simulink model "LIVA_AUV_SIMULATOR"  (R2023b)
settings: Solver=ode4  StartTime=0.0  StopTime=100  FixedStep=0.001  RelTol=0.01  EnableMultiTasking=on
InitFcn:
  | LIVA_AUV_Simulator_init;
model workspace (MAT data in the model file):
  a = 0.0768559116543
  a1 = 5.09287831845
  b = 2.78447714902
  b1 = 0.0150573456987
  c = 0.222680447107
  c1 = 0.0244981849866
  d = 1.17025942432
  d1 = -0.121090969634
  e = 4
  e1 = -0.000744741765672
  f = 3.22045295126
  f1 = 0.147531958158
  g = 3
  g1 = 9.31921319068e-05
  h = 4
  h1 = -0.000787888183232
  i = 2.39426372075
  i1 = -0.0976897881188
  j = 3
  j1 = 7.29765081481
  k = 2
  k1 = 3.34164431501
  l = -0.0819081975806
  l1 = 4.85550524224
  m = -0.0907196254339
  m1 = 2.91684244028
  n = 1.20537954163
  n1 = 9.00648148706
  o = 1.92822193114
  o1 = 2.79427167815
  p = 1.9547800679
  p1 = 9.64465760947
  r = 2
  r1 = 9.85880905818
  s = 0.00182097897058
  s1 = 6.72892013716
values from neighbouring files (symbols this model uses):
  alfa = 1.1    [LIVA_AUV_Simulator_init.m]
  B = 114.8*pk    (= 149.24)    [LIVA_AUV_Simulator_init.m]
  Hybrid_pKd = 1.9282219311449538    (= 1.92822193114)    [LIVA_AUV_Simulator_init.m]
  Hybrid_pKi = 1.205379541632126    (= 1.20537954163)    [LIVA_AUV_Simulator_init.m]
  Hybrid_pKp = -0.090719625433908213    (= -0.0907196254339)    [LIVA_AUV_Simulator_init.m]
  Hybrid_rKd = -0.0819081975805605    (= -0.0819081975806)    [LIVA_AUV_Simulator_init.m]
  Hybrid_rKi = 2    [LIVA_AUV_Simulator_init.m]
  Hybrid_rKp = 3    [LIVA_AUV_Simulator_init.m]
  Hybrid_xalfa = 5.092878318451735    (= 5.09287831845)    [LIVA_AUV_Simulator_init.m]
  Hybrid_xbeta = 0.024498184986623803    (= 0.0244981849866)    [LIVA_AUV_Simulator_init.m]
  Hybrid_xKd = 0.22268044710682114    (= 0.222680447107)    [LIVA_AUV_Simulator_init.m]
  Hybrid_xKi = 2.7844771490230995    (= 2.78447714902)    [LIVA_AUV_Simulator_init.m]
  Hybrid_xKp = 0.076855911654313547    (= 0.0768559116543)    [LIVA_AUV_Simulator_init.m]
  Hybrid_yalfa = -0.12109096963388193    (= -0.121090969634)    [LIVA_AUV_Simulator_init.m]
  Hybrid_ybeta = 0.14753195815811565    (= 0.147531958158)    [LIVA_AUV_Simulator_init.m]
  Hybrid_yKd = 3.2204529512582094    (= 3.22045295126)    [LIVA_AUV_Simulator_init.m]
  Hybrid_yKi = 4    [LIVA_AUV_Simulator_init.m]
  Hybrid_yKp = 1.1702594243169564    (= 1.17025942432)    [LIVA_AUV_Simulator_init.m]
  Hybrid_ywKd = 0.001820978970578287    (= 0.00182097897058)    [LIVA_AUV_Simulator_init.m]
  Hybrid_ywKi = 2    [LIVA_AUV_Simulator_init.m]
  Hybrid_ywKp = 1.9547800678980167    (= 1.9547800679)    [LIVA_AUV_Simulator_init.m]
  Hybrid_zalfa = 0.000093192131906777681    (= 9.31921319068e-05)    [LIVA_AUV_Simulator_init.m]
  Hybrid_zbeta = -0.097689788118772547    (= -0.0976897881188)    [LIVA_AUV_Simulator_init.m]
  Hybrid_zKd = 2.3942637207502    (= 2.39426372075)    [LIVA_AUV_Simulator_init.m]
  Hybrid_zKi = 4    [LIVA_AUV_Simulator_init.m]
  Hybrid_zKp = 3    [LIVA_AUV_Simulator_init.m]
  iPID_pKd = 0.00013750228463629022    (= 0.000137502284636)    [LIVA_AUV_Simulator_init.m]
  iPID_pKi = 0.031254576821627369    (= 0.0312545768216)    [LIVA_AUV_Simulator_init.m]
  iPID_pKp = 0    [LIVA_AUV_Simulator_init.m]
  iPID_rKd = 2    [LIVA_AUV_Simulator_init.m]
  iPID_rKi = 9.65529148649622E-19    (= 9.6552914865e-19)    [LIVA_AUV_Simulator_init.m]
  iPID_rKp = 3    [LIVA_AUV_Simulator_init.m]
  iPID_xKd = 0    [LIVA_AUV_Simulator_init.m]
  iPID_xKi = 1.1219546659293831    (= 1.12195466593)    [LIVA_AUV_Simulator_init.m]
  iPID_xKp = 0.018002365678869262    (= 0.0180023656789)    [LIVA_AUV_Simulator_init.m]
  iPID_yKd = 3.4277809029094881E-18    (= 3.42778090291e-18)    [LIVA_AUV_Simulator_init.m]
  iPID_yKi = 0.13401348623396903    (= 0.134013486234)    [LIVA_AUV_Simulator_init.m]
  iPID_yKp = 3    [LIVA_AUV_Simulator_init.m]
  iPID_ywKd = 0.62280020767048139    (= 0.62280020767)    [LIVA_AUV_Simulator_init.m]
  iPID_ywKi = 2    [LIVA_AUV_Simulator_init.m]
  iPID_ywKp = 0.87058892280816969    (= 0.870588922808)    [LIVA_AUV_Simulator_init.m]
  iPID_zKd = 0.00075053756185264819    (= 0.000750537561853)    [LIVA_AUV_Simulator_init.m]
  iPID_zKi = 3.5484685597653076    (= 3.54846855977)    [LIVA_AUV_Simulator_init.m]
  iPID_zKp = 0.26825539985723995    (= 0.268255399857)    [LIVA_AUV_Simulator_init.m]
  Ix = 0.16*pk    (= 0.208)    [LIVA_AUV_Simulator_init.m]
  Iy = 0.16*pk    (= 0.208)    [LIVA_AUV_Simulator_init.m]
  Iz = 0.16*pk    (= 0.208)    [LIVA_AUV_Simulator_init.m]
  Kc = 20*eye(6)    [LIVA_AUV_Simulator_init.m]
  Kp = 11.7*pk    (= 15.21)    [LIVA_AUV_Simulator_init.m]
  Kpdot = 0*pk    (= 0)    [LIVA_AUV_Simulator_init.m]
  Kpp = 1.55*pk    (= 2.015)    [LIVA_AUV_Simulator_init.m]
  Mq = 15*pk    (= 19.5)    [LIVA_AUV_Simulator_init.m]
  Mqdot = 0.0023*pk    (= 0.00299)    [LIVA_AUV_Simulator_init.m]
  Mqq = 1.55*pk    (= 2.015)    [LIVA_AUV_Simulator_init.m]
  Nr = 30*pk    (= 39)    [LIVA_AUV_Simulator_init.m]
  Nrdot = 0.0023*pk    (= 0.00299)    [LIVA_AUV_Simulator_init.m]
  Nrr = 1.55*pk    (= 2.015)    [LIVA_AUV_Simulator_init.m]
  PID_pKd = -0.04940918869876651    (= -0.0494091886988)    [LIVA_AUV_Simulator_init.m]
  PID_pKi = 2    [LIVA_AUV_Simulator_init.m]
  PID_pKp = -0.39327079611315297    (= -0.393270796113)    [LIVA_AUV_Simulator_init.m]
  PID_rKd = -0.054985573360707168    (= -0.0549855733607)    [LIVA_AUV_Simulator_init.m]
  PID_rKi = 0.001    [LIVA_AUV_Simulator_init.m]
  PID_rKp = -0.040345732248197354    (= -0.0403457322482)    [LIVA_AUV_Simulator_init.m]
  PID_xKd = 4    [LIVA_AUV_Simulator_init.m]
  PID_xKi = 4    [LIVA_AUV_Simulator_init.m]
  PID_xKp = 3    [LIVA_AUV_Simulator_init.m]
  PID_yKd = 3.1154066328676535    (= 3.11540663287)    [LIVA_AUV_Simulator_init.m]
  PID_yKi = 4    [LIVA_AUV_Simulator_init.m]
  PID_yKp = 3    [LIVA_AUV_Simulator_init.m]
  PID_ywKd = 0.89665765450717427    (= 0.896657654507)    [LIVA_AUV_Simulator_init.m]
  PID_ywKi = -0.006253695766722793    (= -0.00625369576672)    [LIVA_AUV_Simulator_init.m]
  PID_ywKp = 0.98566932171151178    (= 0.985669321712)    [LIVA_AUV_Simulator_init.m]
  PID_zKd = 0.01813689620732389    (= 0.0181368962073)    [LIVA_AUV_Simulator_init.m]
  PID_zKi = 4    [LIVA_AUV_Simulator_init.m]
  PID_zKp = 3    [LIVA_AUV_Simulator_init.m]
  Tmax = 40    [LIVA_AUV_Simulator_init.m]
  Ts_controller = 0.001    [LIVA_AUV_Simulator_init.m]
  twodof_palfa = 0.25    [LIVA_AUV_Simulator_init.m]
  twodof_pbeta = 0.12    [LIVA_AUV_Simulator_init.m]
  twodof_pKd = 0.095424714936744218    (= 0.0954247149367)    [LIVA_AUV_Simulator_init.m]
  twodof_pKi = 0.13825854798036114    (= 0.13825854798)    [LIVA_AUV_Simulator_init.m]
  twodof_pKp = 0.11369893762575015    (= 0.113698937626)    [LIVA_AUV_Simulator_init.m]
  twodof_ralfa = 0.19999999999999798    (= 0.2)    [LIVA_AUV_Simulator_init.m]
  twodof_rbeta = 0.20000000000000065    (= 0.2)    [LIVA_AUV_Simulator_init.m]
  twodof_rKd = 0.53578437965746184    (= 0.535784379657)    [LIVA_AUV_Simulator_init.m]
  twodof_rKi = 1.1506401605012322    (= 1.1506401605)    [LIVA_AUV_Simulator_init.m]
  twodof_rKp = 2.9999790377213507    (= 2.99997903772)    [LIVA_AUV_Simulator_init.m]
  twodof_xalfa = 0.30234710594262    (= 0.302347105943)    [LIVA_AUV_Simulator_init.m]
  twodof_xbeta = 1.7366690704427536    (= 1.73666907044)    [LIVA_AUV_Simulator_init.m]
  twodof_xKd = 0.97271920084965735    (= 0.97271920085)    [LIVA_AUV_Simulator_init.m]
  twodof_xKi = 3.9943078181304963    (= 3.99430781813)    [LIVA_AUV_Simulator_init.m]
  twodof_xKp = 0.28411216909151349    (= 0.284112169092)    [LIVA_AUV_Simulator_init.m]
  twodof_yalfa = 0.10435250246875363    (= 0.104352502469)    [LIVA_AUV_Simulator_init.m]
  twodof_ybeta = 0.005650227565256156    (= 0.00565022756526)    [LIVA_AUV_Simulator_init.m]
  twodof_yKd = 0.18997113533365648    (= 0.189971135334)    [LIVA_AUV_Simulator_init.m]
  twodof_yKi = 3.9999790377213498    (= 3.99997903772)    [LIVA_AUV_Simulator_init.m]
  twodof_yKp = 0.063666271676642031    (= 0.0636662716766)    [LIVA_AUV_Simulator_init.m]
  twodof_ywalfa = -4.2798991350061177    (= -4.27989913501)    [LIVA_AUV_Simulator_init.m]
  twodof_ywbeta = 0.35373480857737255    (= 0.353734808577)    [LIVA_AUV_Simulator_init.m]
  twodof_ywKd = 1.0659867557210738    (= 1.06598675572)    [LIVA_AUV_Simulator_init.m]
  twodof_ywKi = 0.00008440390384513819    (= 8.44039038451e-05)    [LIVA_AUV_Simulator_init.m]
  twodof_ywKp = 0.28527888951964514    (= 0.28527888952)    [LIVA_AUV_Simulator_init.m]
  twodof_zalfa = 0.00008034865340691478    (= 8.03486534069e-05)    [LIVA_AUV_Simulator_init.m]
  twodof_zbeta = 0.32801506093302246    (= 0.328015060933)    [LIVA_AUV_Simulator_init.m]
  twodof_zKd = 2.2289396936947683    (= 2.22893969369)    [LIVA_AUV_Simulator_init.m]
  twodof_zKi = 3.8840765857077431    (= 3.88407658571)    [LIVA_AUV_Simulator_init.m]
  twodof_zKp = 2.9999790377213507    (= 2.99997903772)    [LIVA_AUV_Simulator_init.m]
  W = 112.8*pk    (= 146.64)    [LIVA_AUV_Simulator_init.m]
  xb = 0    [LIVA_AUV_Simulator_init.m]
  xg = 0    [LIVA_AUV_Simulator_init.m]
  Xu = 26*pk    (= 33.8)    [LIVA_AUV_Simulator_init.m]
  Xudot = 10.6505*pk    (= 13.84565)    [LIVA_AUV_Simulator_init.m]
  Xuu = 18.18*pk    (= 23.634)    [LIVA_AUV_Simulator_init.m]
  yb = 0    [LIVA_AUV_Simulator_init.m]
  yg = 0    [LIVA_AUV_Simulator_init.m]
  Yv = 30*pk    (= 39)    [LIVA_AUV_Simulator_init.m]
  Yvdot = 11.9247*pk    (= 15.50211)    [LIVA_AUV_Simulator_init.m]
  Yvv = 21.66*pk    (= 28.158)    [LIVA_AUV_Simulator_init.m]
  zb = 0    [LIVA_AUV_Simulator_init.m]
  zg = 0.02    [LIVA_AUV_Simulator_init.m]
  ... (+3 more)
undefined symbols (not defined in the file or in its folder): DiscIntNeverNeededParam, gray, sigbuilder_block
libraries: slpidlib x29, eeGeneralControl x19, pid_lib x6, simulink x4, sim3dlib x4
(part 5 of 6)

== system LIVA_AUV_SIMULATOR/6DOF CONTROL/i-PID Controler/i-PID Controller  ==
  note: iPID Control Signals
  note: Error Signals
  Body Frame Reference Trajectory : Inport
  Error Signals : Inport  Port=2
  Body Frame Positions : Inport  Port=3
  Calculation : Subsystem
  Demux : Demux  Outputs=6
  Mux2 : Mux  Inputs=6
  PID Controller : pid_lib/PID Controller  Controller=PID  Form=Parallel  TimeDomain=Discrete-time  UseExternalTs=off  SampleTime=-1  IntegratorMethod=Forward Euler  FilterMethod=Forward Euler  ControllerParametersSource=internal  P=iPID_xKp  I=iPID_xKi  D=iPID_xKd  UseFilter=on  N=1  TunerSelectOption=Transfer Function Based (PID Tuner App)  InitialConditionSource=internal  InitialConditionForIntegrator=0  InitialConditionForFilter=0  DifferentiatorICPrevScaledInput=0  ExternalReset=none  TrackingMode=off  Kt=1  LimitOutput=on  SatLimitsSource=internal  UpperSaturationLimit=inf  LowerSaturationLimit=-inf  LinearizeAsGain=on  AntiWindupMode=back-calculation  Kb=1  POutMin=[]  POutMax=[]  IOutMin=[]  IOutMax=[]  DOutMin=[]  DOutMax=[]  NOutMin=[]  NOutMax=[]  SumOutMin=[]  SumOutMax=[]  SaturationOutMin=[]  SaturationOutMax=[]  PParamMin=[]  PParamMax=[]  IParamMin=[]  IParamMax=[]  DParamMin=[]  DParamMax=[]  NParamMin=[]  NParamMax=[]  KbParamMin=[]  KbParamMax=[]  KtParamMin=[]  KtParamMax=[]  KbOutMin=[]  KbOutMax=[]  KtOutMin=[]  KtOutMax=[]  IntegratorOutMin=[]  IntegratorOutMax=[]  FilterOutMin=[]  FilterOutMax=[]  SumI1OutMin=[]  SumI1OutMax=[]  SumI2OutMin=[]  SumI2OutMax=[]  SumI3OutMin=[]  SumI3OutMax=[]  SumI4OutMin=[]  SumI4OutMax=[]  SumDOutMin=[]  SumDOutMax=[]  DifferentiatorOutMin=[]  DifferentiatorOutMax=[]  FilterDiffOutCoefMin=[]  FilterDiffOutCoefMax=[]  ReciprocalOutMin=[]  ReciprocalOutMax=[]  SumDenOutMin=[]  SumDenOutMax=[]  SumNumOutMin=[]  SumNumOutMax=[]  DivideOutMin=[]  DivideOutMax=[]  UdiffTsProdOutMin=[]  UdiffTsProdOutMax=[]  NTsProdOutMin=[]  NTsProdOutMax=[]  UintegralTsProdOutMin=[]  UintegralTsProdOutMax=[]  UngainTsProdOutMin=[]  UngainTsProdOutMax=[]  IntegratorContinuousStateAttributes=''  IntegratorStateMustResolveToSignalObject=off  IntegratorRTWStateStorageClass=Auto  FilterContinuousStateAttributes=''  FilterStateMustResolveToSignalObject=off  FilterRTWStateStorageClass=Auto  ParallelPVariant=InternalParameters  IdealPVariant=Disabled  IVariant=InternalParameters  DVariant=InternalParameters  IntegratorVariant=Discrete  SatVariant=Enabled  AWVariant=BackCalculation  PCopyVariant=Disabled  TRVariant=Disabled  FdbkBlocksVariant=Forward  IdealPFdbkVariant=Disabled  SatFdbkVariant=Disabled  DerivativeFilterVariant=ForwardEulerFilter  NVariant=InternalParameters  NCopyVariant=Disabled  FilterICVariant=InternalICsFilter  IntegratorICVariant=InternalICs  ExternalResetVariant=Disabled  TRSumVariant=Passthrough  SumFdbkVariant=Disabled  SumVariant=Sum_PID  TsampFilterVariant=InternalTs  TsampNgainVariant=Passthrough  TsampIntegralVariant=Passthrough  ExternalSaturationOutDataTypeStr=Inherit: Same as second input
  PID Controller1 : pid_lib/PID Controller  Controller=PID  Form=Parallel  TimeDomain=Discrete-time  UseExternalTs=off  SampleTime=-1  IntegratorMethod=Forward Euler  FilterMethod=Forward Euler  ControllerParametersSource=internal  P=iPID_yKp  I=iPID_yKi  D=iPID_yKd  UseFilter=on  N=3  TunerSelectOption=Transfer Function Based (PID Tuner App)  InitialConditionSource=internal  InitialConditionForIntegrator=0  InitialConditionForFilter=0  DifferentiatorICPrevScaledInput=0  ExternalReset=none  TrackingMode=off  Kt=1  LimitOutput=on  SatLimitsSource=internal  UpperSaturationLimit=inf  LowerSaturationLimit=-inf  LinearizeAsGain=on  AntiWindupMode=back-calculation  Kb=1  POutMin=[]  POutMax=[]  IOutMin=[]  IOutMax=[]  DOutMin=[]  DOutMax=[]  NOutMin=[]  NOutMax=[]  SumOutMin=[]  SumOutMax=[]  SaturationOutMin=[]  SaturationOutMax=[]  PParamMin=[]  PParamMax=[]  IParamMin=[]  IParamMax=[]  DParamMin=[]  DParamMax=[]  NParamMin=[]  NParamMax=[]  KbParamMin=[]  KbParamMax=[]  KtParamMin=[]  KtParamMax=[]  KbOutMin=[]  KbOutMax=[]  KtOutMin=[]  KtOutMax=[]  IntegratorOutMin=[]  IntegratorOutMax=[]  FilterOutMin=[]  FilterOutMax=[]  SumI1OutMin=[]  SumI1OutMax=[]  SumI2OutMin=[]  SumI2OutMax=[]  SumI3OutMin=[]  SumI3OutMax=[]  SumI4OutMin=[]  SumI4OutMax=[]  SumDOutMin=[]  SumDOutMax=[]  DifferentiatorOutMin=[]  DifferentiatorOutMax=[]  FilterDiffOutCoefMin=[]  FilterDiffOutCoefMax=[]  ReciprocalOutMin=[]  ReciprocalOutMax=[]  SumDenOutMin=[]  SumDenOutMax=[]  SumNumOutMin=[]  SumNumOutMax=[]  DivideOutMin=[]  DivideOutMax=[]  UdiffTsProdOutMin=[]  UdiffTsProdOutMax=[]  NTsProdOutMin=[]  NTsProdOutMax=[]  UintegralTsProdOutMin=[]  UintegralTsProdOutMax=[]  UngainTsProdOutMin=[]  UngainTsProdOutMax=[]  IntegratorContinuousStateAttributes=''  IntegratorStateMustResolveToSignalObject=off  IntegratorRTWStateStorageClass=Auto  FilterContinuousStateAttributes=''  FilterStateMustResolveToSignalObject=off  FilterRTWStateStorageClass=Auto  ParallelPVariant=InternalParameters  IdealPVariant=Disabled  IVariant=InternalParameters  DVariant=InternalParameters  IntegratorVariant=Discrete  SatVariant=Enabled  AWVariant=BackCalculation  PCopyVariant=Disabled  TRVariant=Disabled  FdbkBlocksVariant=Forward  IdealPFdbkVariant=Disabled  SatFdbkVariant=Disabled  DerivativeFilterVariant=ForwardEulerFilter  NVariant=InternalParameters  NCopyVariant=Disabled  FilterICVariant=InternalICsFilter  IntegratorICVariant=InternalICs  ExternalResetVariant=Disabled  TRSumVariant=Passthrough  SumFdbkVariant=Disabled  SumVariant=Sum_PID  TsampFilterVariant=InternalTs  TsampNgainVariant=Passthrough  TsampIntegralVariant=Passthrough  ExternalSaturationOutDataTypeStr=Inherit: Same as second input
  PID Controller2 : pid_lib/PID Controller  Controller=PID  Form=Parallel  TimeDomain=Discrete-time  UseExternalTs=off  SampleTime=-1  IntegratorMethod=Forward Euler  FilterMethod=Forward Euler  ControllerParametersSource=internal  P=iPID_zKp  I=iPID_zKi  D=iPID_zKd  UseFilter=on  N=1  TunerSelectOption=Transfer Function Based (PID Tuner App)  InitialConditionSource=internal  InitialConditionForIntegrator=0  InitialConditionForFilter=0  DifferentiatorICPrevScaledInput=0  ExternalReset=none  TrackingMode=off  Kt=1  LimitOutput=on  SatLimitsSource=internal  UpperSaturationLimit=inf  LowerSaturationLimit=-inf  LinearizeAsGain=on  AntiWindupMode=back-calculation  Kb=1  POutMin=[]  POutMax=[]  IOutMin=[]  IOutMax=[]  DOutMin=[]  DOutMax=[]  NOutMin=[]  NOutMax=[]  SumOutMin=[]  SumOutMax=[]  SaturationOutMin=[]  SaturationOutMax=[]  PParamMin=[]  PParamMax=[]  IParamMin=[]  IParamMax=[]  DParamMin=[]  DParamMax=[]  NParamMin=[]  NParamMax=[]  KbParamMin=[]  KbParamMax=[]  KtParamMin=[]  KtParamMax=[]  KbOutMin=[]  KbOutMax=[]  KtOutMin=[]  KtOutMax=[]  IntegratorOutMin=[]  IntegratorOutMax=[]  FilterOutMin=[]  FilterOutMax=[]  SumI1OutMin=[]  SumI1OutMax=[]  SumI2OutMin=[]  SumI2OutMax=[]  SumI3OutMin=[]  SumI3OutMax=[]  SumI4OutMin=[]  SumI4OutMax=[]  SumDOutMin=[]  SumDOutMax=[]  DifferentiatorOutMin=[]  DifferentiatorOutMax=[]  FilterDiffOutCoefMin=[]  FilterDiffOutCoefMax=[]  ReciprocalOutMin=[]  ReciprocalOutMax=[]  SumDenOutMin=[]  SumDenOutMax=[]  SumNumOutMin=[]  SumNumOutMax=[]  DivideOutMin=[]  DivideOutMax=[]  UdiffTsProdOutMin=[]  UdiffTsProdOutMax=[]  NTsProdOutMin=[]  NTsProdOutMax=[]  UintegralTsProdOutMin=[]  UintegralTsProdOutMax=[]  UngainTsProdOutMin=[]  UngainTsProdOutMax=[]  IntegratorContinuousStateAttributes=''  IntegratorStateMustResolveToSignalObject=off  IntegratorRTWStateStorageClass=Auto  FilterContinuousStateAttributes=''  FilterStateMustResolveToSignalObject=off  FilterRTWStateStorageClass=Auto  ParallelPVariant=InternalParameters  IdealPVariant=Disabled  IVariant=InternalParameters  DVariant=InternalParameters  IntegratorVariant=Discrete  SatVariant=Enabled  AWVariant=BackCalculation  PCopyVariant=Disabled  TRVariant=Disabled  FdbkBlocksVariant=Forward  IdealPFdbkVariant=Disabled  SatFdbkVariant=Disabled  DerivativeFilterVariant=ForwardEulerFilter  NVariant=InternalParameters  NCopyVariant=Disabled  FilterICVariant=InternalICsFilter  IntegratorICVariant=InternalICs  ExternalResetVariant=Disabled  TRSumVariant=Passthrough  SumFdbkVariant=Disabled  SumVariant=Sum_PID  TsampFilterVariant=InternalTs  TsampNgainVariant=Passthrough  TsampIntegralVariant=Passthrough  ExternalSaturationOutDataTypeStr=Inherit: Same as second input
  PID Controller3 : pid_lib/PID Controller  Controller=PID  Form=Parallel  TimeDomain=Discrete-time  UseExternalTs=off  SampleTime=-1  IntegratorMethod=Forward Euler  FilterMethod=Forward Euler  ControllerParametersSource=internal  P=iPID_rKp  I=iPID_rKi  D=iPID_rKd  UseFilter=on  N=1  TunerSelectOption=Transfer Function Based (PID Tuner App)  InitialConditionSource=internal  InitialConditionForIntegrator=0  InitialConditionForFilter=0  DifferentiatorICPrevScaledInput=0  ExternalReset=none  TrackingMode=off  Kt=1  LimitOutput=on  SatLimitsSource=internal  UpperSaturationLimit=inf  LowerSaturationLimit=-inf  LinearizeAsGain=on  AntiWindupMode=back-calculation  Kb=1  POutMin=[]  POutMax=[]  IOutMin=[]  IOutMax=[]  DOutMin=[]  DOutMax=[]  NOutMin=[]  NOutMax=[]  SumOutMin=[]  SumOutMax=[]  SaturationOutMin=[]  SaturationOutMax=[]  PParamMin=[]  PParamMax=[]  IParamMin=[]  IParamMax=[]  DParamMin=[]  DParamMax=[]  NParamMin=[]  NParamMax=[]  KbParamMin=[]  KbParamMax=[]  KtParamMin=[]  KtParamMax=[]  KbOutMin=[]  KbOutMax=[]  KtOutMin=[]  KtOutMax=[]  IntegratorOutMin=[]  IntegratorOutMax=[]  FilterOutMin=[]  FilterOutMax=[]  SumI1OutMin=[]  SumI1OutMax=[]  SumI2OutMin=[]  SumI2OutMax=[]  SumI3OutMin=[]  SumI3OutMax=[]  SumI4OutMin=[]  SumI4OutMax=[]  SumDOutMin=[]  SumDOutMax=[]  DifferentiatorOutMin=[]  DifferentiatorOutMax=[]  FilterDiffOutCoefMin=[]  FilterDiffOutCoefMax=[]  ReciprocalOutMin=[]  ReciprocalOutMax=[]  SumDenOutMin=[]  SumDenOutMax=[]  SumNumOutMin=[]  SumNumOutMax=[]  DivideOutMin=[]  DivideOutMax=[]  UdiffTsProdOutMin=[]  UdiffTsProdOutMax=[]  NTsProdOutMin=[]  NTsProdOutMax=[]  UintegralTsProdOutMin=[]  UintegralTsProdOutMax=[]  UngainTsProdOutMin=[]  UngainTsProdOutMax=[]  IntegratorContinuousStateAttributes=''  IntegratorStateMustResolveToSignalObject=off  IntegratorRTWStateStorageClass=Auto  FilterContinuousStateAttributes=''  FilterStateMustResolveToSignalObject=off  FilterRTWStateStorageClass=Auto  ParallelPVariant=InternalParameters  IdealPVariant=Disabled  IVariant=InternalParameters  DVariant=InternalParameters  IntegratorVariant=Discrete  SatVariant=Enabled  AWVariant=BackCalculation  PCopyVariant=Disabled  TRVariant=Disabled  FdbkBlocksVariant=Forward  IdealPFdbkVariant=Disabled  SatFdbkVariant=Disabled  DerivativeFilterVariant=ForwardEulerFilter  NVariant=InternalParameters  NCopyVariant=Disabled  FilterICVariant=InternalICsFilter  IntegratorICVariant=InternalICs  ExternalResetVariant=Disabled  TRSumVariant=Passthrough  SumFdbkVariant=Disabled  SumVariant=Sum_PID  TsampFilterVariant=InternalTs  TsampNgainVariant=Passthrough  TsampIntegralVariant=Passthrough  ExternalSaturationOutDataTypeStr=Inherit: Same as second input
  PID Controller4 : pid_lib/PID Controller  Controller=PID  Form=Parallel  TimeDomain=Discrete-time  UseExternalTs=off  SampleTime=-1  IntegratorMethod=Forward Euler  FilterMethod=Forward Euler  ControllerParametersSource=internal  P=iPID_pKp  I=iPID_pKi  D=iPID_pKd  UseFilter=on  N=1  TunerSelectOption=Transfer Function Based (PID Tuner App)  InitialConditionSource=internal  InitialConditionForIntegrator=0  InitialConditionForFilter=0  DifferentiatorICPrevScaledInput=0  ExternalReset=none  TrackingMode=off  Kt=1  LimitOutput=on  SatLimitsSource=internal  UpperSaturationLimit=inf  LowerSaturationLimit=-inf  LinearizeAsGain=on  AntiWindupMode=back-calculation  Kb=1  POutMin=[]  POutMax=[]  IOutMin=[]  IOutMax=[]  DOutMin=[]  DOutMax=[]  NOutMin=[]  NOutMax=[]  SumOutMin=[]  SumOutMax=[]  SaturationOutMin=[]  SaturationOutMax=[]  PParamMin=[]  PParamMax=[]  IParamMin=[]  IParamMax=[]  DParamMin=[]  DParamMax=[]  NParamMin=[]  NParamMax=[]  KbParamMin=[]  KbParamMax=[]  KtParamMin=[]  KtParamMax=[]  KbOutMin=[]  KbOutMax=[]  KtOutMin=[]  KtOutMax=[]  IntegratorOutMin=[]  IntegratorOutMax=[]  FilterOutMin=[]  FilterOutMax=[]  SumI1OutMin=[]  SumI1OutMax=[]  SumI2OutMin=[]  SumI2OutMax=[]  SumI3OutMin=[]  SumI3OutMax=[]  SumI4OutMin=[]  SumI4OutMax=[]  SumDOutMin=[]  SumDOutMax=[]  DifferentiatorOutMin=[]  DifferentiatorOutMax=[]  FilterDiffOutCoefMin=[]  FilterDiffOutCoefMax=[]  ReciprocalOutMin=[]  ReciprocalOutMax=[]  SumDenOutMin=[]  SumDenOutMax=[]  SumNumOutMin=[]  SumNumOutMax=[]  DivideOutMin=[]  DivideOutMax=[]  UdiffTsProdOutMin=[]  UdiffTsProdOutMax=[]  NTsProdOutMin=[]  NTsProdOutMax=[]  UintegralTsProdOutMin=[]  UintegralTsProdOutMax=[]  UngainTsProdOutMin=[]  UngainTsProdOutMax=[]  IntegratorContinuousStateAttributes=''  IntegratorStateMustResolveToSignalObject=off  IntegratorRTWStateStorageClass=Auto  FilterContinuousStateAttributes=''  FilterStateMustResolveToSignalObject=off  FilterRTWStateStorageClass=Auto  ParallelPVariant=InternalParameters  IdealPVariant=Disabled  IVariant=InternalParameters  DVariant=InternalParameters  IntegratorVariant=Discrete  SatVariant=Enabled  AWVariant=BackCalculation  PCopyVariant=Disabled  TRVariant=Disabled  FdbkBlocksVariant=Forward  IdealPFdbkVariant=Disabled  SatFdbkVariant=Disabled  DerivativeFilterVariant=ForwardEulerFilter  NVariant=InternalParameters  NCopyVariant=Disabled  FilterICVariant=InternalICsFilter  IntegratorICVariant=InternalICs  ExternalResetVariant=Disabled  TRSumVariant=Passthrough  SumFdbkVariant=Disabled  SumVariant=Sum_PID  TsampFilterVariant=InternalTs  TsampNgainVariant=Passthrough  TsampIntegralVariant=Passthrough  ExternalSaturationOutDataTypeStr=Inherit: Same as second input
  PID Controller5 : pid_lib/PID Controller  Controller=PID  Form=Parallel  TimeDomain=Discrete-time  UseExternalTs=off  SampleTime=-1  IntegratorMethod=Forward Euler  FilterMethod=Forward Euler  ControllerParametersSource=internal  P=iPID_ywKp  I=iPID_ywKi  D=iPID_ywKd  UseFilter=on  N=1  TunerSelectOption=Transfer Function Based (PID Tuner App)  InitialConditionSource=internal  InitialConditionForIntegrator=0  InitialConditionForFilter=0  DifferentiatorICPrevScaledInput=0  ExternalReset=none  TrackingMode=off  Kt=1  LimitOutput=on  SatLimitsSource=internal  UpperSaturationLimit=inf  LowerSaturationLimit=-inf  LinearizeAsGain=on  AntiWindupMode=back-calculation  Kb=1  POutMin=[]  POutMax=[]  IOutMin=[]  IOutMax=[]  DOutMin=[]  DOutMax=[]  NOutMin=[]  NOutMax=[]  SumOutMin=[]  SumOutMax=[]  SaturationOutMin=[]  SaturationOutMax=[]  PParamMin=[]  PParamMax=[]  IParamMin=[]  IParamMax=[]  DParamMin=[]  DParamMax=[]  NParamMin=[]  NParamMax=[]  KbParamMin=[]  KbParamMax=[]  KtParamMin=[]  KtParamMax=[]  KbOutMin=[]  KbOutMax=[]  KtOutMin=[]  KtOutMax=[]  IntegratorOutMin=[]  IntegratorOutMax=[]  FilterOutMin=[]  FilterOutMax=[]  SumI1OutMin=[]  SumI1OutMax=[]  SumI2OutMin=[]  SumI2OutMax=[]  SumI3OutMin=[]  SumI3OutMax=[]  SumI4OutMin=[]  SumI4OutMax=[]  SumDOutMin=[]  SumDOutMax=[]  DifferentiatorOutMin=[]  DifferentiatorOutMax=[]  FilterDiffOutCoefMin=[]  FilterDiffOutCoefMax=[]  ReciprocalOutMin=[]  ReciprocalOutMax=[]  SumDenOutMin=[]  SumDenOutMax=[]  SumNumOutMin=[]  SumNumOutMax=[]  DivideOutMin=[]  DivideOutMax=[]  UdiffTsProdOutMin=[]  UdiffTsProdOutMax=[]  NTsProdOutMin=[]  NTsProdOutMax=[]  UintegralTsProdOutMin=[]  UintegralTsProdOutMax=[]  UngainTsProdOutMin=[]  UngainTsProdOutMax=[]  IntegratorContinuousStateAttributes=''  IntegratorStateMustResolveToSignalObject=off  IntegratorRTWStateStorageClass=Auto  FilterContinuousStateAttributes=''  FilterStateMustResolveToSignalObject=off  FilterRTWStateStorageClass=Auto  ParallelPVariant=InternalParameters  IdealPVariant=Disabled  IVariant=InternalParameters  DVariant=InternalParameters  IntegratorVariant=Discrete  SatVariant=Enabled  AWVariant=BackCalculation  PCopyVariant=Disabled  TRVariant=Disabled  FdbkBlocksVariant=Forward  IdealPFdbkVariant=Disabled  SatFdbkVariant=Disabled  DerivativeFilterVariant=ForwardEulerFilter  NVariant=InternalParameters  NCopyVariant=Disabled  FilterICVariant=InternalICsFilter  IntegratorICVariant=InternalICs  ExternalResetVariant=Disabled  TRSumVariant=Passthrough  SumFdbkVariant=Disabled  SumVariant=Sum_PID  TsampFilterVariant=InternalTs  TsampNgainVariant=Passthrough  TsampIntegralVariant=Passthrough  ExternalSaturationOutDataTypeStr=Inherit: Same as second input
  iPID Control Signals : Outport  VectorParamsAs1DForOutWhenUnconnected=off
  wires:
  Body Frame Reference Trajectory/1 -> Calculation/1(Body Frame Reference Trajectory)
  Body Frame Positions/1 -> Calculation/3(Body Frame Positions)
  Calculation/1(IPI Controller Outputs) -> iPID Control Signals/1
  PID Controller3/1 -> Mux2/4
  Error Signals/1 -> Demux/1
  Demux/5 -> PID Controller4/1
  PID Controller2/1 -> Mux2/3
  PID Controller1/1 -> Mux2/2
  Demux/4 -> PID Controller3/1
  Demux/1 -> PID Controller/1
  Mux2/1 -> Calculation/2(PI Controller Outputs)  "PI Controller Outputs"
  PID Controller5/1 -> Mux2/6
  PID Controller4/1 -> Mux2/5
  Demux/3 -> PID Controller2/1
  Demux/2 -> PID Controller1/1
  Demux/6 -> PID Controller5/1
  PID Controller/1 -> Mux2/1

== system LIVA_AUV_SIMULATOR/Evaluation & Visualization/Variant Subsystem/3D Unreal Engine ==
  Visualization : Inport
  Constant : Constant  Value=[1 1 1]
  Demux : Demux  Outputs=2
  Simulation 3D Actor Transform Set : sim3dlib/Simulation 3D Actor Transform Set  Priority=-1  ActorTag=Sub1  NumberOfParts=1  CustNumOfParts=3  Translation=[0 0 0]  Rotation=[0 0 0]  Scale=[1 1 1]  Ts=-1  aMode=2
  Simulation 3D Camera Get : sim3dlib/Simulation 3D Camera Get  Priority=1  sensorTag=Sim3dSensor3  sensorId=3  sensorName=Sim3dSensor3  vehTagList={'Scene Origin'}  vehTag=Scene Origin  mountLoc=Origin  offsetFlag=on  tmountOffset=[6.5, 13.5, 12]  rmountOffset=[0, 28, 225]  HorizontalResolution=1280  VerticalResolution=720  HorizontalFOV=60  SampleTime=-1  mountPoint=[6.5 -13.5 12]  mountOrientation=[0 -28 -225]  aMode=2  ID=3
  Simulation 3D Scene Configuration : sim3dlib/Simulation 3D Scene Configuration  Priority=0  ProjectFormat=Unreal Editor  SceneDesc=Straight road  ProjectName=C:\MATLAB\toolbox\shared\sim3d_projects\automotive_project\UE4\WindowsNoEditor\VehicleSimulation.exe  ScenePath=/Game/Maps/HwStrght  UEProjPath=D:\UE\projects\MyProject77\MyProject77.uproject  EnableOpenDRIVE=off  vehTagList={'Scene Origin'}  vehTag=Scene Origin  OpVisEn=off  Ts=0.01  EnableWindow=on  EnableRemoteAccess=off  EnableWeather=off  SunAltitude=40.0  SunAzimuth=90  clouds=10  wind=1  fog=0  rain=0  EnableGeospatial=off  OriginHeight=200  OriginLatitude=40.744652  OriginLongitude=-73.988864  MapStyle=Aerial  AdditionalAssetIDs=[]  UseAdvancedSunSky=off  SolarTime=11  TimeZone=-5  Day=21  Month=9  Year=2022  UseDaylightSavingTime=on  DSTStartDay=10  DSTStartMonth=3  DSTEndDay=3  DSTEndMonth=11  DSTSwitchHour=2  sensorTag=MainCamera1  sensorId=1  sensorName=MainCamera1  mountLoc=Origin  offsetFlag=off  tmountOffset=[0, 0, 0]  rmountOffset=[0, 0, 0]  HorizontalResolution=1280  VerticalResolution=720  HorizontalFOV=60  mountPoint=[0 0 0]  mountOrientation=[0 0 0]  aMode=2  ID=1  GeoTrigger=Inactive
  Subsystem : Subsystem
  Subsystem1 : Subsystem
  Video Viewer : VideoViewer  colormapValue=gray(256)  FigPos=[624 1037 1296 929]
  wires:
  Subsystem1/1(Out1) -> Simulation 3D Actor Transform Set/2
  Constant/1 -> Simulation 3D Actor Transform Set/3
  Demux/2 -> Subsystem1/1(In1)
  Demux/1 -> Subsystem/1(In1)
  Subsystem/1(Out1) -> Simulation 3D Actor Transform Set/1
  Simulation 3D Camera Get/1 -> Video Viewer/1
  Visualization/1 -> Demux/1

== system LIVA_AUV_SIMULATOR/Evaluation & Visualization/Variant Subsystem/Simulink Scopes ==
  Visualization : Inport

== system LIVA_AUV_SIMULATOR/6DOF CONTROL/2 DoF i-PID Controller/ i-PID Feedback Controller /Calculation ==
  Body Frame Reference Trajectory : Inport
  PI Controller Outputs : Inport  Port=2
  Body Frame Positions : Inport  Port=3
  Divide : Product  Inputs=*/
  Divide1 : Product  Inputs=**
  Divide2 : Product  Inputs=*/
  Filtered Derivative (Discrete or Continuous){,1..3} (4 alike) : eeGeneralControl/Filtered Derivative (Discrete or Continuous)  K=1  T=1  B=inf  A=-inf  minRatio=10  init_option=Inherited from block input  x0=0  Ts=-1
  Sum : Sum  Inputs=|+-
  Sum1 : Sum  Inputs=|+-
  Sum2 : Sum  Inputs=|++
  Unit Delay : UnitDelay  SampleTime=-1  HasFrameUpgradeWarning=on
  a : Constant  Value=alfa
  IPI Controller Outputs : Outport
  wires:
  a/1 -> Divide1/2, Divide/2, Divide2/2
  Divide/1 -> Sum/2
  Divide1/1 -> Sum1/2
  Sum1/1 -> Divide/1  "F"
  Unit Delay/1 -> Divide1/1
  Filtered Derivative (Discrete or Continuous)1/1 -> Sum/1
  Body Frame Reference Trajectory/1 -> Filtered Derivative (Discrete or Continuous)/1
  PI Controller Outputs/1 -> Sum2/2
  Sum/1 -> Divide2/1
  Divide2/1 -> Sum2/1
  Sum2/1 -> Unit Delay/1, IPI Controller Outputs/1
  Body Frame Positions/1 -> Filtered Derivative (Discrete or Continuous)2/1
  Filtered Derivative (Discrete or Continuous)3/1 -> Sum1/1
  Filtered Derivative (Discrete or Continuous)/1 -> Filtered Derivative (Discrete or Continuous)1/1
  Filtered Derivative (Discrete or Continuous)2/1 -> Filtered Derivative (Discrete or Continuous)3/1

== system LIVA_AUV_SIMULATOR/6DOF CONTROL/Hybrid i-PID Controller/2-DoF i-PID Position Controller/Feedback i-PID Controller  ==
  note: iPID Control Signals
  note: Error Signals
  Body Frame Reference Trajectory : Inport
  Error Signals : Inport  Port=2
  Body Frame Positions : Inport  Port=3
  Calculation : Subsystem
  Demux : Demux  Outputs=3
  Mux2 : Mux  Inputs=3
  PID Controller : slpidlib/PID Controller  Controller=PID  Form=Parallel  TimeDomain=Discrete-time  UseExternalTs=off  SampleTime=Ts_controller  IntegratorMethod=Forward Euler  FilterMethod=Forward Euler  ControllerParametersSource=internal  P=Hybrid_xKp  I=Hybrid_xKi  UseKiTs=off  D=Hybrid_xKd  N=0.8  UseFilter=on  TunerSelectOption=Transfer Function Based (PID Tuner App)  InitialConditionSource=internal  InitialConditionForIntegrator=0  InitialConditionForFilter=0  DifferentiatorICPrevScaledInput=0  ExternalReset=none  TrackingMode=off  Kt=1  LimitOutput=on  SatLimitsSource=internal  UpperSaturationLimit=inf  LowerSaturationLimit=-inf  LinearizeAsGain=on  AntiWindupMode=back-calculation  Kb=1  LimitIntegrator=off  UpperIntegratorSaturationLimit=inf  LowerIntegratorSaturationLimit=-inf  POutMin=[]  POutMax=[]  IOutMin=[]  IOutMax=[]  DOutMin=[]  DOutMax=[]  NOutMin=[]  NOutMax=[]  SumOutMin=[]  SumOutMax=[]  SaturationOutMin=[]  SaturationOutMax=[]  PParamMin=[]  PParamMax=[]  IParamMin=[]  IParamMax=[]  DParamMin=[]  DParamMax=[]  NParamMin=[]  NParamMax=[]  KbParamMin=[]  KbParamMax=[]  KtParamMin=[]  KtParamMax=[]  KbOutMin=[]  KbOutMax=[]  KtOutMin=[]  KtOutMax=[]  IntegratorOutMin=[]  IntegratorOutMax=[]  FilterOutMin=[]  FilterOutMax=[]  SumI1OutMin=[]  SumI1OutMax=[]  SumI2OutMin=[]  SumI2OutMax=[]  SumI3OutMin=[]  SumI3OutMax=[]  SumI4OutMin=[]  SumI4OutMax=[]  SumDOutMin=[]  SumDOutMax=[]  DifferentiatorOutMin=[]  DifferentiatorOutMax=[]  FilterDiffOutCoefMin=[]  FilterDiffOutCoefMax=[]  ReciprocalOutMin=[]  ReciprocalOutMax=[]  SumDenOutMin=[]  SumDenOutMax=[]  SumNumOutMin=[]  SumNumOutMax=[]  DivideOutMin=[]  DivideOutMax=[]  UdiffTsProdOutMin=[]  UdiffTsProdOutMax=[]  NTsProdOutMin=[]  NTsProdOutMax=[]  UintegralTsProdOutMin=[]  UintegralTsProdOutMax=[]  UngainTsProdOutMin=[]  UngainTsProdOutMax=[]  ClampingZeroOutDataTypeStr=Inherit: Inherit via back propagation  ClampingZeroOutMin=[]  ClampingZeroOutMax=[]  FilterDenConstantOutDataTypeStr=Inherit: Inherit via back propagation  FilterDenConstantOutMin=[]  FilterDenConstantOutMax=[]  PCopyOutDataTypeStr=Inherit: Inherit via back propagation  PCopyOutMin=[]  PCopyOutMax=[]  NCopyOutDataTypeStr=Inherit: Inherit via back propagation  NCopyOutMin=[]  NCopyOutMax=[]  IntegratorContinuousStateAttributes=''  IntegratorStateMustResolveToSignalObject=off  IntegratorRTWStateStorageClass=Auto  FilterContinuousStateAttributes=''  FilterStateMustResolveToSignalObject=off  FilterRTWStateStorageClass=Auto  ParallelPVariant=InternalParameters  IdealPVariant=Disabled  IVariant=InternalParameters  DVariant=InternalParameters  IntegratorVariant=Discrete  SatVariant=Enabled  AWVariant=BackCalculation  PCopyVariant=Disabled  TRVariant=Disabled  FdbkBlocksVariant=Forward  IdealPFdbkVariant=Disabled  SatFdbkVariant=Disabled  DerivativeFilterVariant=ForwardEulerFilter  NVariant=InternalParameters  NCopyVariant=Disabled  FilterICVariant=InternalICsFilter  IntegratorICVariant=InternalICs  ExternalResetVariant=Disabled  TRSumVariant=Passthrough  SumFdbkVariant=Disabled  SumVariant=Sum_PID  TsampFilterVariant=InternalTs  TsampNgainVariant=Passthrough  TsampIntegralVariant=Disabled_SignalSpec  ExternalSaturationOutDataTypeStr=Inherit: Same as second input
  PID Controller1 : slpidlib/PID Controller  Controller=PID  Form=Parallel  TimeDomain=Discrete-time  UseExternalTs=off  SampleTime=Ts_controller  IntegratorMethod=Forward Euler  FilterMethod=Forward Euler  ControllerParametersSource=internal  P=Hybrid_yKp  I=Hybrid_yKi  UseKiTs=off  D=Hybrid_yKd  N=0.8  UseFilter=on  TunerSelectOption=Transfer Function Based (PID Tuner App)  InitialConditionSource=internal  InitialConditionForIntegrator=0  InitialConditionForFilter=0  DifferentiatorICPrevScaledInput=0  ExternalReset=none  TrackingMode=off  Kt=1  LimitOutput=on  SatLimitsSource=internal  UpperSaturationLimit=inf  LowerSaturationLimit=-inf  LinearizeAsGain=on  AntiWindupMode=back-calculation  Kb=1  LimitIntegrator=off  UpperIntegratorSaturationLimit=inf  LowerIntegratorSaturationLimit=-inf  POutMin=[]  POutMax=[]  IOutMin=[]  IOutMax=[]  DOutMin=[]  DOutMax=[]  NOutMin=[]  NOutMax=[]  SumOutMin=[]  SumOutMax=[]  SaturationOutMin=[]  SaturationOutMax=[]  PParamMin=[]  PParamMax=[]  IParamMin=[]  IParamMax=[]  DParamMin=[]  DParamMax=[]  NParamMin=[]  NParamMax=[]  KbParamMin=[]  KbParamMax=[]  KtParamMin=[]  KtParamMax=[]  KbOutMin=[]  KbOutMax=[]  KtOutMin=[]  KtOutMax=[]  IntegratorOutMin=[]  IntegratorOutMax=[]  FilterOutMin=[]  FilterOutMax=[]  SumI1OutMin=[]  SumI1OutMax=[]  SumI2OutMin=[]  SumI2OutMax=[]  SumI3OutMin=[]  SumI3OutMax=[]  SumI4OutMin=[]  SumI4OutMax=[]  SumDOutMin=[]  SumDOutMax=[]  DifferentiatorOutMin=[]  DifferentiatorOutMax=[]  FilterDiffOutCoefMin=[]  FilterDiffOutCoefMax=[]  ReciprocalOutMin=[]  ReciprocalOutMax=[]  SumDenOutMin=[]  SumDenOutMax=[]  SumNumOutMin=[]  SumNumOutMax=[]  DivideOutMin=[]  DivideOutMax=[]  UdiffTsProdOutMin=[]  UdiffTsProdOutMax=[]  NTsProdOutMin=[]  NTsProdOutMax=[]  UintegralTsProdOutMin=[]  UintegralTsProdOutMax=[]  UngainTsProdOutMin=[]  UngainTsProdOutMax=[]  ClampingZeroOutDataTypeStr=Inherit: Inherit via back propagation  ClampingZeroOutMin=[]  ClampingZeroOutMax=[]  FilterDenConstantOutDataTypeStr=Inherit: Inherit via back propagation  FilterDenConstantOutMin=[]  FilterDenConstantOutMax=[]  PCopyOutDataTypeStr=Inherit: Inherit via back propagation  PCopyOutMin=[]  PCopyOutMax=[]  NCopyOutDataTypeStr=Inherit: Inherit via back propagation  NCopyOutMin=[]  NCopyOutMax=[]  IntegratorContinuousStateAttributes=''  IntegratorStateMustResolveToSignalObject=off  IntegratorRTWStateStorageClass=Auto  FilterContinuousStateAttributes=''  FilterStateMustResolveToSignalObject=off  FilterRTWStateStorageClass=Auto  ParallelPVariant=InternalParameters  IdealPVariant=Disabled  IVariant=InternalParameters  DVariant=InternalParameters  IntegratorVariant=Discrete  SatVariant=Enabled  AWVariant=BackCalculation  PCopyVariant=Disabled  TRVariant=Disabled  FdbkBlocksVariant=Forward  IdealPFdbkVariant=Disabled  SatFdbkVariant=Disabled  DerivativeFilterVariant=ForwardEulerFilter  NVariant=InternalParameters  NCopyVariant=Disabled  FilterICVariant=InternalICsFilter  IntegratorICVariant=InternalICs  ExternalResetVariant=Disabled  TRSumVariant=Passthrough  SumFdbkVariant=Disabled  SumVariant=Sum_PID  TsampFilterVariant=InternalTs  TsampNgainVariant=Passthrough  TsampIntegralVariant=Disabled_SignalSpec  ExternalSaturationOutDataTypeStr=Inherit: Same as second input
  PID Controller2 : slpidlib/PID Controller  Controller=PID  Form=Parallel  TimeDomain=Discrete-time  UseExternalTs=off  SampleTime=Ts_controller  IntegratorMethod=Forward Euler  FilterMethod=Forward Euler  ControllerParametersSource=internal  P=Hybrid_zKp  I=Hybrid_zKi  UseKiTs=off  D=Hybrid_zKd  N=0.8  UseFilter=on  TunerSelectOption=Transfer Function Based (PID Tuner App)  InitialConditionSource=internal  InitialConditionForIntegrator=0  InitialConditionForFilter=0  DifferentiatorICPrevScaledInput=0  ExternalReset=none  TrackingMode=off  Kt=1  LimitOutput=on  SatLimitsSource=internal  UpperSaturationLimit=inf  LowerSaturationLimit=-inf  LinearizeAsGain=on  AntiWindupMode=back-calculation  Kb=1  LimitIntegrator=off  UpperIntegratorSaturationLimit=inf  LowerIntegratorSaturationLimit=-inf  POutMin=[]  POutMax=[]  IOutMin=[]  IOutMax=[]  DOutMin=[]  DOutMax=[]  NOutMin=[]  NOutMax=[]  SumOutMin=[]  SumOutMax=[]  SaturationOutMin=[]  SaturationOutMax=[]  PParamMin=[]  PParamMax=[]  IParamMin=[]  IParamMax=[]  DParamMin=[]  DParamMax=[]  NParamMin=[]  NParamMax=[]  KbParamMin=[]  KbParamMax=[]  KtParamMin=[]  KtParamMax=[]  KbOutMin=[]  KbOutMax=[]  KtOutMin=[]  KtOutMax=[]  IntegratorOutMin=[]  IntegratorOutMax=[]  FilterOutMin=[]  FilterOutMax=[]  SumI1OutMin=[]  SumI1OutMax=[]  SumI2OutMin=[]  SumI2OutMax=[]  SumI3OutMin=[]  SumI3OutMax=[]  SumI4OutMin=[]  SumI4OutMax=[]  SumDOutMin=[]  SumDOutMax=[]  DifferentiatorOutMin=[]  DifferentiatorOutMax=[]  FilterDiffOutCoefMin=[]  FilterDiffOutCoefMax=[]  ReciprocalOutMin=[]  ReciprocalOutMax=[]  SumDenOutMin=[]  SumDenOutMax=[]  SumNumOutMin=[]  SumNumOutMax=[]  DivideOutMin=[]  DivideOutMax=[]  UdiffTsProdOutMin=[]  UdiffTsProdOutMax=[]  NTsProdOutMin=[]  NTsProdOutMax=[]  UintegralTsProdOutMin=[]  UintegralTsProdOutMax=[]  UngainTsProdOutMin=[]  UngainTsProdOutMax=[]  ClampingZeroOutDataTypeStr=Inherit: Inherit via back propagation  ClampingZeroOutMin=[]  ClampingZeroOutMax=[]  FilterDenConstantOutDataTypeStr=Inherit: Inherit via back propagation  FilterDenConstantOutMin=[]  FilterDenConstantOutMax=[]  PCopyOutDataTypeStr=Inherit: Inherit via back propagation  PCopyOutMin=[]  PCopyOutMax=[]  NCopyOutDataTypeStr=Inherit: Inherit via back propagation  NCopyOutMin=[]  NCopyOutMax=[]  IntegratorContinuousStateAttributes=''  IntegratorStateMustResolveToSignalObject=off  IntegratorRTWStateStorageClass=Auto  FilterContinuousStateAttributes=''  FilterStateMustResolveToSignalObject=off  FilterRTWStateStorageClass=Auto  ParallelPVariant=InternalParameters  IdealPVariant=Disabled  IVariant=InternalParameters  DVariant=InternalParameters  IntegratorVariant=Discrete  SatVariant=Enabled  AWVariant=BackCalculation  PCopyVariant=Disabled  TRVariant=Disabled  FdbkBlocksVariant=Forward  IdealPFdbkVariant=Disabled  SatFdbkVariant=Disabled  DerivativeFilterVariant=ForwardEulerFilter  NVariant=InternalParameters  NCopyVariant=Disabled  FilterICVariant=InternalICsFilter  IntegratorICVariant=InternalICs  ExternalResetVariant=Disabled  TRSumVariant=Passthrough  SumFdbkVariant=Disabled  SumVariant=Sum_PID  TsampFilterVariant=InternalTs  TsampNgainVariant=Passthrough  TsampIntegralVariant=Disabled_SignalSpec  ExternalSaturationOutDataTypeStr=Inherit: Same as second input
  iPID Control Signals : Outport  VectorParamsAs1DForOutWhenUnconnected=off
  wires:
  Body Frame Reference Trajectory/1 -> Calculation/1(Body Frame Reference Trajectory)
  Body Frame Positions/1 -> Calculation/3(Body Frame Positions)
  Calculation/1(IPI Controller Outputs) -> iPID Control Signals/1
  Error Signals/1 -> Demux/1
  PID Controller2/1 -> Mux2/3
  PID Controller1/1 -> Mux2/2
  Demux/1 -> PID Controller/1
  Mux2/1 -> Calculation/2(PI Controller Outputs)  "PI Controller Outputs"
  Demux/3 -> PID Controller2/1
  Demux/2 -> PID Controller1/1
  PID Controller/1 -> Mux2/1
